simulink model "simu_2nd_ordre_ericc3"  (R2016b)
settings: Solver=VariableStepAuto  StartTime=0.0  StopTime=10.0  RelTol=1e-3
values from neighbouring files (symbols this model uses):
  tau = tpic-Tp/2    [ide_temporelle.m]    (also in test.m = 3)
  w0 = wp2/sqrt(1-xi^2)    [ide_temporelle.m]
  xi = abs(log(D1))/(sqrt(pi^2+(log(D1))^2))    [ide_temporelle.m]
settings Model: Creator=emiliendurif  LastModifiedBy=emiliendurif

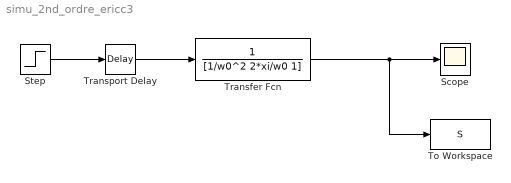
== system simu_2nd_ordre_ericc3 ==
  Scope : Scope
  Step : Step  Time=0  After=30  SampleTime=0
  To Workspace : ToWorkspace  VariableName=S  SaveFormat=Timeseries  SampleTime=-1
  Transfer Fcn : TransferFcn  Denominator=[1/w0^2 2*xi/w0 1]
  Transport Delay : TransportDelay  DelayTime=tau
  wires:
  Step/1 -> Transport Delay/1
  Transfer Fcn/1 -> To Workspace/1, Scope/1
  Transport Delay/1 -> Transfer Fcn/1
